simulink model "pfb_fir_generic_async_test_sim4"  (R2012b)
settings: Solver=VariableStepDiscrete  StartTime=0.0  StopTime=10.0  RelTol=1e-3
model workspace (MAT data in the model file):
  synci = [0 1 2 3 4 5 6 7 8 9 10 11 ... (131074 elements, 65537x2)]
  din0 = [0 1 2 3 4 5 6 7 8 9 10 11 ... (16386 elements, 8193x2)]
  din1 = [0 1 2 3 4 5 6 7 8 9 10 11 ... (16386 elements, 8193x2)]
  din2 = [0 1 2 3 4 5 6 7 8 9 10 11 ... (16386 elements, 8193x2)]
  din3 = [0 1 2 3 4 5 6 7 8 9 10 11 ... (16386 elements, 8193x2)]
  din4 = [0 1 2 3 4 5 6 7 8 9 10 11 ... (16386 elements, 8193x2)]
  din5 = [0 1 2 3 4 5 6 7 8 9 10 11 ... (16386 elements, 8193x2)]
  din6 = [0 1 2 3 4 5 6 7 8 9 10 11 ... (16386 elements, 8193x2)]
  din7 = [0 1 2 3 4 5 6 7 8 9 10 11 ... (16386 elements, 8193x2)]
  dvalid = [0 1 2 3 4 5 6 7 8 9 10 11 ... (131072 elements, 65536x2)]
libraries: xbsIndex_r4 x3718, casper_library_delays x1
(part 10 of 18)

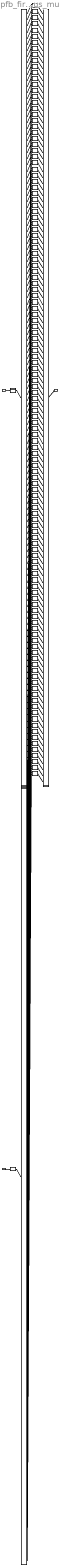
== system pfb_fir_generic_async_test_sim4/pfb_fir_generic/pfb_fir_taps/bus_mult ==
  a : Inport
  b : Inport  Port=2
  a*b_bussify : Subsystem  AncestorBlock=casper_library_flow_control/bus_create  mask(bus_create){inputNum=128}
      mask prompts: inputNum "Number of inputs:"
      mask init:
      | bus_create_init(gcb,...
      |     'inputNum', inputNum);
  a_debus : Subsystem  AncestorBlock=casper_library_flow_control/bus_expand  mask(bus_expand){mode=divisions of arbitrary size, outputNum=1, outputWidth=[10 10 10 10 10 10 10 10 10 10 10 10 10 10 10 10 10 10 10 10 10 10 10 10 10 10 10 10 10 10 10 10 10 10 10 10 10 10 10 10 10 10 10 10 10 10 10 10 10 10 10 10 10 10 10 10 10 10 10 10 10 10 10 10 10 10 10 10 10 10 10 10 10 10 10 10 10 10 10 10 10 10 10 10 10 10 10 10 10 10 10 10 10 10 10 10 10 10 10 10 10 10 10 10 10 10 10 10 10 10 10 10 10 10 10 10 10 10 10 10 10 10 10 10 10 10 10 10], outputBinaryPt=[9 9 9 9 9 9 9 9 9 9 9 9 9 9 9 9 9 9 9 9 9 9 9 9 9 9 9 9 9 9 9 9 9 9 9 9 9 9 9 9 9 9 9 9 9 9 9 9 9 9 9 9 9 9 9 9 9 9 9 9 9 9 9 9 9 9 9 9 9 9 9 9 9 9 9 9 9 9 9 9 9 9 9 9 9 9 9 9 9 9 9 9 9 9 9 9 9 9 9 9 9 9 9 9 9 9 9 9 9 9 9 9 9 9 9 9 9 9 9 9 9 9 9 9 9 9 9 9], outputArithmeticType=[1 1 1 1 1 1 1 1 1 1 1 1 1 1 1 1 1 1 1 1 1 1 1 1 1 1 1 1 1 1 1 1 1 1 1 1 1 1 1 1 1 1 1 1 1 1 1 1 1 1 1 1 1 1 1 1 1 1 1 1 1 1 1 1 1 1 1 1 1 1 1 1 1 1 1 1 1 1 1 1 1 1 1 1 1 1 1 1 1 1 1 1 1 1 1 1 1 1 1 1 1 1 1 1 1 1 1 1 1 1 1 1 1 1 1 1 1 1 1 1 1 1 1 1 1 1 1 1], show_format=on, outputToWorkspace=off, variablePrefix=, outputToModelAsWell=on}
      mask prompts: outputNum "Number of outputs:"; outputWidth "Output width [msb ... lsb]:"; outputBinaryPt "Output binary point position [msb ... lsb]:"; outputArithmeticType "Output arithmetic type (ufix=0, fix=1, bool=2) [msb ... lsb]:"; show_format "Print format string?"; outputToWorkspace "Output to workspace?"; variablePrefix "Variable name prefix:"; outputToModelAsWell "Output to model as well?"
      mask help:
      | Expands a 'bus' made using a bus_create or Xilinx
      | concat block.
      | The input will be divided into the specified number
      | of outputs with the specified arithmetic types.
      | Divisions are made from most significant bit.
      mask init: same as pfb_fir_generic_async_test_sim4/pfb_fir_generic/bus_expand
      settings: AttributesFormatString=128 outputs: f10.9,f10.9,f10.9,f10.9,f10.9,f10.9,f10.9,f10.9,f10.9,f10.9,f10.9,f10.9,f10.9,f10.9,f10.9,f10.9,f10.9,f10.9,f10.9,f10.9,f10.9,f10.9,f10.9,f10.9,f10.9,f10.9,f10.9,f10.9,f10.9,f10.9,f10.9,f10.9,f10.9,f10.9,f10.9,f10.9,f10.9,f10.9,f10.9,f10.9,f10.9,f10.9,f10.9,f10.9,f10.9,f10.9,f10.9,f10.9,f10.9,f10.9,f10.9,f10.9,f10.9,f10.9,f10.9,f10.9,f10.9,f10.9,f10.9,f10.9,f10.9,f10.9,f10.9,f10.9,f10.9,f10.9,f10.9,f10.9,f10.9,f10.9,f10.9,f10.9,f10.9,f10.9,f10.9,f10.9,f10.9,f10.9,f10.9,f10.9,f10.9,f10.9,f10.9,f10.9,f10.9,f10.9,f10.9,f10.9,f10.9,f10.9,f10.9,f10.9,f10.9,f10.9,f10.9,f10.9,f10.9,f10.9,f10.9,f10.9,f10.9,f10.9,f10.9,f10.9,f10.9,f10.9,f10.9,f10.9,f10.9,f10.9,f10.9,f10.9,f10.9,f10.9,f10.9,f10.9,f10.9,f10.9,f10.9,f10.9,f10.9,f10.9,f10.9,f10.9,f10.9,f10.9,f10.9,f10.9,
      mask TypeOptions mode: divisions of equal size | divisions of arbitrary size
      mask Callback mode: bus_expand_callback();
      mask Callback outputWidth: bus_expand_callback();
      mask Callback outputToWorkspace: bus_expand_callback();
  b_debus : Subsystem  AncestorBlock=casper_library_flow_control/bus_expand  mask(bus_expand){mode=divisions of arbitrary size, outputNum=1, outputWidth=[18 18 18 18 18 18 18 18 18 18 18 18 18 18 18 18 18 18 18 18 18 18 18 18 18 18 18 18 18 18 18 18 18 18 18 18 18 18 18 18 18 18 18 18 18 18 18 18 18 18 18 18 18 18 18 18 18 18 18 18 18 18 18 18 18 18 18 18 18 18 18 18 18 18 18 18 18 18 18 18 18 18 18 18 18 18 18 18 18 18 18 18 18 18 18 18 18 18 18 18 18 18 18 18 18 18 18 18 18 18 18 18 18 18 18 18 18 18 18 18 18 18 18 18 18 18 18 18], outputBinaryPt=[17 17 17 17 17 17 17 17 17 17 17 17 17 17 17 17 17 17 17 17 17 17 17 17 17 17 17 17 17 17 17 17 17 17 17 17 17 17 17 17 17 17 17 17 17 17 17 17 17 17 17 17 17 17 17 17 17 17 17 17 17 17 17 17 17 17 17 17 17 17 17 17 17 17 17 17 17 17 17 17 17 17 17 17 17 17 17 17 17 17 17 17 17 17 17 17 17 17 17 17 17 17 17 17 17 17 17 17 17 17 17 17 17 17 17 17 17 17 17 17 17 17 17 17 17 17 17 17], outputArithmeticType=[1 1 1 1 1 1 1 1 1 1 1 1 1 1 1 1 1 1 1 1 1 1 1 1 1 1 1 1 1 1 1 1 1 1 1 1 1 1 1 1 1 1 1 1 1 1 1 1 1 1 1 1 1 1 1 1 1 1 1 1 1 1 1 1 1 1 1 1 1 1 1 1 1 1 1 1 1 1 1 1 1 1 1 1 1 1 1 1 1 1 1 1 1 1 1 1 1 1 1 1 1 1 1 1 1 1 1 1 1 1 1 1 1 1 1 1 1 1 1 1 1 1 1 1 1 1 1 1], show_format=on, outputToWorkspace=off, variablePrefix=, outputToModelAsWell=on}
      mask prompts: outputNum "Number of outputs:"; outputWidth "Output width [msb ... lsb]:"; outputBinaryPt "Output binary point position [msb ... lsb]:"; outputArithmeticType "Output arithmetic type (ufix=0, fix=1, bool=2) [msb ... lsb]:"; show_format "Print format string?"; outputToWorkspace "Output to workspace?"; variablePrefix "Variable name prefix:"; outputToModelAsWell "Output to model as well?"
      mask help:
      | Expands a 'bus' made using a bus_create or Xilinx
      | concat block.
      | The input will be divided into the specified number
      | of outputs with the specified arithmetic types.
      | Divisions are made from most significant bit.
      mask init: same as pfb_fir_generic_async_test_sim4/pfb_fir_generic/bus_expand
      settings: AttributesFormatString=128 outputs: f18.17,f18.17,f18.17,f18.17,f18.17,f18.17,f18.17,f18.17,f18.17,f18.17,f18.17,f18.17,f18.17,f18.17,f18.17,f18.17,f18.17,f18.17,f18.17,f18.17,f18.17,f18.17,f18.17,f18.17,f18.17,f18.17,f18.17,f18.17,f18.17,f18.17,f18.17,f18.17,f18.17,f18.17,f18.17,f18.17,f18.17,f18.17,f18.17,f18.17,f18.17,f18.17,f18.17,f18.17,f18.17,f18.17,f18.17,f18.17,f18.17,f18.17,f18.17,f18.17,f18.17,f18.17,f18.17,f18.17,f18.17,f18.17,f18.17,f18.17,f18.17,f18.17,f18.17,f18.17,f18.17,f18.17,f18.17,f18.17,f18.17,f18.17,f18.17,f18.17,f18.17,f18.17,f18.17,f18.17,f18.17,f18.17,f18.17,f18.17,f18.17,f18.17,f18.17,f18.17,f18.17,f18.17,f18.17,f18.17,f18.17,f18.17,f18.17,f18.17,f18.17,f18.17,f18.17,f18.17,f18.17,f18.17,f18.17,f18.17,f18.17,f18.17,f18.17,f18.17,f18.17,f18.17,f18.17,f18.17,f18.17,f18.17,f18.17,f18.17,f18.17,f18.17,f18.17,f18.17,f18.17,f18.17,f18.17,f18.17,f18.17,f18.17,f18.17,f18.17,f18.17,f18.17,f18.17,f18.17,
      mask TypeOptions mode: divisions of equal size | divisions of arbitrary size
      mask Callback mode: bus_expand_callback();
      mask Callback outputWidth: bus_expand_callback();
      mask Callback outputToWorkspace: bus_expand_callback();
  mult{1..128} (128 alike) : xbsIndex_r4/Mult  precision=User Defined  arith_type="Signed  (2's comp)"  n_bits=28  bin_pt=26  quantization=Truncate  overflow=Wrap  en=off  latency=mult_latency  dbl_ovrd=off  use_behavioral_HDL=on  opt=Speed  use_embedded=off  optimum_pipeline=off  pipeline=on  use_rpm=on  placement_style=Triangular  block_type=mult
  repa : Subsystem  AncestorBlock=casper_library_bus/bus_replicate  mask(bus_replicate){replication=1, latency=0, misc=off, implementation=core}
      mask prompts: replication "replication factor"; misc "misc support"; implementation "delay implementation"
      mask help: Output bus formed by replicating input bus a number of times
      mask init:
      | bus_replicate_init(gcb, ...
      |     'replication', replication, ...
      |     'latency', latency, ...
      |     'implementation', implementation, ...
      |     'misc', misc);
      mask TypeOptions implementation: core | behavioral
  repb : Subsystem  AncestorBlock=casper_library_bus/bus_replicate  mask(bus_replicate){replication=1, latency=0, misc=off, implementation=core}
      mask prompts: replication "replication factor"; misc "misc support"; implementation "delay implementation"
      mask help: Output bus formed by replicating input bus a number of times
      mask init:
      | bus_replicate_init(gcb, ...
      |     'replication', replication, ...
      |     'latency', latency, ...
      |     'implementation', implementation, ...
      |     'misc', misc);
      mask TypeOptions implementation: core | behavioral
  a*b : Outport
  wires:
  a/1 -> repa/1(in)
  b/1 -> repb/1(in)
  repa/1(out) -> a_debus/1(bus_in)
  repb/1(out) -> b_debus/1(bus_in)
  a_debus/1(msb_out128) -> mult1/1
  b_debus/1(msb_out128) -> mult1/2
  a_debus/2(out127) -> mult2/1
  b_debus/2(out127) -> mult2/2
  a_debus/3(out126) -> mult3/1
  b_debus/3(out126) -> mult3/2
  a_debus/4(out125) -> mult4/1
  b_debus/4(out125) -> mult4/2
  a_debus/5(out124) -> mult5/1
  b_debus/5(out124) -> mult5/2
  a_debus/6(out123) -> mult6/1
  b_debus/6(out123) -> mult6/2
  a_debus/7(out122) -> mult7/1
  b_debus/7(out122) -> mult7/2
  a_debus/8(out121) -> mult8/1
  b_debus/8(out121) -> mult8/2
  a_debus/9(out120) -> mult9/1
  b_debus/9(out120) -> mult9/2
  a_debus/10(out119) -> mult10/1
  b_debus/10(out119) -> mult10/2
  a_debus/11(out118) -> mult11/1
  b_debus/11(out118) -> mult11/2
  a_debus/12(out117) -> mult12/1
  b_debus/12(out117) -> mult12/2
  a_debus/13(out116) -> mult13/1
  b_debus/13(out116) -> mult13/2
  a_debus/14(out115) -> mult14/1
  b_debus/14(out115) -> mult14/2
  a_debus/15(out114) -> mult15/1
  b_debus/15(out114) -> mult15/2
  a_debus/16(out113) -> mult16/1
  b_debus/16(out113) -> mult16/2
  a_debus/17(out112) -> mult17/1
  b_debus/17(out112) -> mult17/2
  a_debus/18(out111) -> mult18/1
  b_debus/18(out111) -> mult18/2
  a_debus/19(out110) -> mult19/1
  b_debus/19(out110) -> mult19/2
  a_debus/20(out109) -> mult20/1
  b_debus/20(out109) -> mult20/2
  a_debus/21(out108) -> mult21/1
  b_debus/21(out108) -> mult21/2
  a_debus/22(out107) -> mult22/1
  b_debus/22(out107) -> mult22/2
  a_debus/23(out106) -> mult23/1
  b_debus/23(out106) -> mult23/2
  a_debus/24(out105) -> mult24/1
  b_debus/24(out105) -> mult24/2
  a_debus/25(out104) -> mult25/1
  b_debus/25(out104) -> mult25/2
  a_debus/26(out103) -> mult26/1
  b_debus/26(out103) -> mult26/2
  a_debus/27(out102) -> mult27/1
  b_debus/27(out102) -> mult27/2
  a_debus/28(out101) -> mult28/1
  b_debus/28(out101) -> mult28/2
  a_debus/29(out100) -> mult29/1
  b_debus/29(out100) -> mult29/2
  a_debus/30(out99) -> mult30/1
  b_debus/30(out99) -> mult30/2
  a_debus/31(out98) -> mult31/1
  b_debus/31(out98) -> mult31/2
  a_debus/32(out97) -> mult32/1
  b_debus/32(out97) -> mult32/2
  a_debus/33(out96) -> mult33/1
  b_debus/33(out96) -> mult33/2
  a_debus/34(out95) -> mult34/1
  b_debus/34(out95) -> mult34/2
  a_debus/35(out94) -> mult35/1
  b_debus/35(out94) -> mult35/2
  a_debus/36(out93) -> mult36/1
  b_debus/36(out93) -> mult36/2
  a_debus/37(out92) -> mult37/1
  b_debus/37(out92) -> mult37/2
  a_debus/38(out91) -> mult38/1
  b_debus/38(out91) -> mult38/2
  a_debus/39(out90) -> mult39/1
  b_debus/39(out90) -> mult39/2
  a_debus/40(out89) -> mult40/1
  b_debus/40(out89) -> mult40/2
  a_debus/41(out88) -> mult41/1
  b_debus/41(out88) -> mult41/2
  a_debus/42(out87) -> mult42/1
  b_debus/42(out87) -> mult42/2
  a_debus/43(out86) -> mult43/1
  b_debus/43(out86) -> mult43/2
  a_debus/44(out85) -> mult44/1
  b_debus/44(out85) -> mult44/2
  a_debus/45(out84) -> mult45/1
  b_debus/45(out84) -> mult45/2
  a_debus/46(out83) -> mult46/1
  b_debus/46(out83) -> mult46/2
  a_debus/47(out82) -> mult47/1
  b_debus/47(out82) -> mult47/2
  a_debus/48(out81) -> mult48/1
  b_debus/48(out81) -> mult48/2
  a_debus/49(out80) -> mult49/1
  b_debus/49(out80) -> mult49/2
  a_debus/50(out79) -> mult50/1
  b_debus/50(out79) -> mult50/2
  a_debus/51(out78) -> mult51/1
  b_debus/51(out78) -> mult51/2
  a_debus/52(out77) -> mult52/1
  b_debus/52(out77) -> mult52/2
  a_debus/53(out76) -> mult53/1
  b_debus/53(out76) -> mult53/2
  a_debus/54(out75) -> mult54/1
  b_debus/54(out75) -> mult54/2
  a_debus/55(out74) -> mult55/1
  b_debus/55(out74) -> mult55/2
  a_debus/56(out73) -> mult56/1
  b_debus/56(out73) -> mult56/2
  a_debus/57(out72) -> mult57/1
  b_debus/57(out72) -> mult57/2
  a_debus/58(out71) -> mult58/1
  b_debus/58(out71) -> mult58/2
  a_debus/59(out70) -> mult59/1
  b_debus/59(out70) -> mult59/2
  a_debus/60(out69) -> mult60/1
  b_debus/60(out69) -> mult60/2
  a_debus/61(out68) -> mult61/1
  b_debus/61(out68) -> mult61/2
  a_debus/62(out67) -> mult62/1
  b_debus/62(out67) -> mult62/2
  a_debus/63(out66) -> mult63/1
  b_debus/63(out66) -> mult63/2
  a_debus/64(out65) -> mult64/1
  b_debus/64(out65) -> mult64/2
  a_debus/65(out64) -> mult65/1
  b_debus/65(out64) -> mult65/2
  a_debus/66(out63) -> mult66/1
  b_debus/66(out63) -> mult66/2
  a_debus/67(out62) -> mult67/1
  b_debus/67(out62) -> mult67/2
  a_debus/68(out61) -> mult68/1
  b_debus/68(out61) -> mult68/2
  a_debus/69(out60) -> mult69/1
  b_debus/69(out60) -> mult69/2
  a_debus/70(out59) -> mult70/1
  b_debus/70(out59) -> mult70/2
  a_debus/71(out58) -> mult71/1
  b_debus/71(out58) -> mult71/2
  a_debus/72(out57) -> mult72/1
  b_debus/72(out57) -> mult72/2
  a_debus/73(out56) -> mult73/1
  b_debus/73(out56) -> mult73/2
  a_debus/74(out55) -> mult74/1
  b_debus/74(out55) -> mult74/2
  a_debus/75(out54) -> mult75/1
  b_debus/75(out54) -> mult75/2
  a_debus/76(out53) -> mult76/1
  b_debus/76(out53) -> mult76/2
  a_debus/77(out52) -> mult77/1
  b_debus/77(out52) -> mult77/2
  a_debus/78(out51) -> mult78/1
  b_debus/78(out51) -> mult78/2
  a_debus/79(out50) -> mult79/1
  b_debus/79(out50) -> mult79/2
  a_debus/80(out49) -> mult80/1
  b_debus/80(out49) -> mult80/2
  a_debus/81(out48) -> mult81/1
  b_debus/81(out48) -> mult81/2
  a_debus/82(out47) -> mult82/1
  b_debus/82(out47) -> mult82/2
  a_debus/83(out46) -> mult83/1
  b_debus/83(out46) -> mult83/2
  a_debus/84(out45) -> mult84/1
  b_debus/84(out45) -> mult84/2
  a_debus/85(out44) -> mult85/1
  b_debus/85(out44) -> mult85/2
  a_debus/86(out43) -> mult86/1
  b_debus/86(out43) -> mult86/2
  a_debus/87(out42) -> mult87/1
  b_debus/87(out42) -> mult87/2
  a_debus/88(out41) -> mult88/1
  b_debus/88(out41) -> mult88/2
  a_debus/89(out40) -> mult89/1
  b_debus/89(out40) -> mult89/2
  a_debus/90(out39) -> mult90/1
  b_debus/90(out39) -> mult90/2
  a_debus/91(out38) -> mult91/1
  b_debus/91(out38) -> mult91/2
  a_debus/92(out37) -> mult92/1
  b_debus/92(out37) -> mult92/2
  a_debus/93(out36) -> mult93/1
  b_debus/93(out36) -> mult93/2
  a_debus/94(out35) -> mult94/1
  b_debus/94(out35) -> mult94/2
  a_debus/95(out34) -> mult95/1
  b_debus/95(out34) -> mult95/2
  a_debus/96(out33) -> mult96/1
  b_debus/96(out33) -> mult96/2
  a_debus/97(out32) -> mult97/1
  b_debus/97(out32) -> mult97/2
  a_debus/98(out31) -> mult98/1
  b_debus/98(out31) -> mult98/2
  a_debus/99(out30) -> mult99/1
  b_debus/99(out30) -> mult99/2
  a_debus/100(out29) -> mult100/1
  b_debus/100(out29) -> mult100/2
  a_debus/101(out28) -> mult101/1
  b_debus/101(out28) -> mult101/2
  a_debus/102(out27) -> mult102/1
  b_debus/102(out27) -> mult102/2
  a_debus/103(out26) -> mult103/1
  b_debus/103(out26) -> mult103/2
  a_debus/104(out25) -> mult104/1
  b_debus/104(out25) -> mult104/2
  a_debus/105(out24) -> mult105/1
  b_debus/105(out24) -> mult105/2
  a_debus/106(out23) -> mult106/1
  b_debus/106(out23) -> mult106/2
  a_debus/107(out22) -> mult107/1
  b_debus/107(out22) -> mult107/2
  a_debus/108(out21) -> mult108/1
  b_debus/108(out21) -> mult108/2
  a_debus/109(out20) -> mult109/1
  b_debus/109(out20) -> mult109/2
  a_debus/110(out19) -> mult110/1
  b_debus/110(out19) -> mult110/2
  a_debus/111(out18) -> mult111/1
  b_debus/111(out18) -> mult111/2
  a_debus/112(out17) -> mult112/1
  b_debus/112(out17) -> mult112/2
  a_debus/113(out16) -> mult113/1
  b_debus/113(out16) -> mult113/2
  a_debus/114(out15) -> mult114/1
  b_debus/114(out15) -> mult114/2
  a_debus/115(out14) -> mult115/1
  b_debus/115(out14) -> mult115/2
  a_debus/116(out13) -> mult116/1
  b_debus/116(out13) -> mult116/2
  a_debus/117(out12) -> mult117/1
  b_debus/117(out12) -> mult117/2
  a_debus/118(out11) -> mult118/1
  b_debus/118(out11) -> mult118/2
  a_debus/119(out10) -> mult119/1
  b_debus/119(out10) -> mult119/2
  a_debus/120(out9) -> mult120/1
  b_debus/120(out9) -> mult120/2
  a_debus/121(out8) -> mult121/1
  b_debus/121(out8) -> mult121/2
  a_debus/122(out7) -> mult122/1
  b_debus/122(out7) -> mult122/2
  a_debus/123(out6) -> mult123/1
  b_debus/123(out6) -> mult123/2
  a_debus/124(out5) -> mult124/1
  b_debus/124(out5) -> mult124/2
  a_debus/125(out4) -> mult125/1
  b_debus/125(out4) -> mult125/2
  a_debus/126(out3) -> mult126/1
  b_debus/126(out3) -> mult126/2
  a_debus/127(out2) -> mult127/1
  b_debus/127(out2) -> mult127/2
  a_debus/128(lsb_out1) -> mult128/1
  b_debus/128(lsb_out1) -> mult128/2
  mult1/1 -> a*b_bussify/1(in1)
  mult2/1 -> a*b_bussify/2(in2)
  mult3/1 -> a*b_bussify/3(in3)
  mult4/1 -> a*b_bussify/4(in4)
  mult5/1 -> a*b_bussify/5(in5)
  mult6/1 -> a*b_bussify/6(in6)
  mult7/1 -> a*b_bussify/7(in7)
  mult8/1 -> a*b_bussify/8(in8)
  mult9/1 -> a*b_bussify/9(in9)
  mult10/1 -> a*b_bussify/10(in10)
  mult11/1 -> a*b_bussify/11(in11)
  mult12/1 -> a*b_bussify/12(in12)
  mult13/1 -> a*b_bussify/13(in13)
  mult14/1 -> a*b_bussify/14(in14)
  mult15/1 -> a*b_bussify/15(in15)
  mult16/1 -> a*b_bussify/16(in16)
  mult17/1 -> a*b_bussify/17(in17)
  mult18/1 -> a*b_bussify/18(in18)
  mult19/1 -> a*b_bussify/19(in19)
  mult20/1 -> a*b_bussify/20(in20)
  mult21/1 -> a*b_bussify/21(in21)
  mult22/1 -> a*b_bussify/22(in22)
  mult23/1 -> a*b_bussify/23(in23)
  mult24/1 -> a*b_bussify/24(in24)
  mult25/1 -> a*b_bussify/25(in25)
  mult26/1 -> a*b_bussify/26(in26)
  mult27/1 -> a*b_bussify/27(in27)
  mult28/1 -> a*b_bussify/28(in28)
  mult29/1 -> a*b_bussify/29(in29)
  mult30/1 -> a*b_bussify/30(in30)
  mult31/1 -> a*b_bussify/31(in31)
  mult32/1 -> a*b_bussify/32(in32)
  mult33/1 -> a*b_bussify/33(in33)
  mult34/1 -> a*b_bussify/34(in34)
  mult35/1 -> a*b_bussify/35(in35)
  mult36/1 -> a*b_bussify/36(in36)
  mult37/1 -> a*b_bussify/37(in37)
  mult38/1 -> a*b_bussify/38(in38)
  mult39/1 -> a*b_bussify/39(in39)
  mult40/1 -> a*b_bussify/40(in40)
  mult41/1 -> a*b_bussify/41(in41)
  mult42/1 -> a*b_bussify/42(in42)
  mult43/1 -> a*b_bussify/43(in43)
  mult44/1 -> a*b_bussify/44(in44)
  mult45/1 -> a*b_bussify/45(in45)
  mult46/1 -> a*b_bussify/46(in46)
  mult47/1 -> a*b_bussify/47(in47)
  mult48/1 -> a*b_bussify/48(in48)
  mult49/1 -> a*b_bussify/49(in49)
  mult50/1 -> a*b_bussify/50(in50)
  mult51/1 -> a*b_bussify/51(in51)
  mult52/1 -> a*b_bussify/52(in52)
  mult53/1 -> a*b_bussify/53(in53)
  mult54/1 -> a*b_bussify/54(in54)
  mult55/1 -> a*b_bussify/55(in55)
  mult56/1 -> a*b_bussify/56(in56)
  mult57/1 -> a*b_bussify/57(in57)
  mult58/1 -> a*b_bussify/58(in58)
  mult59/1 -> a*b_bussify/59(in59)
  mult60/1 -> a*b_bussify/60(in60)
  mult61/1 -> a*b_bussify/61(in61)
  mult62/1 -> a*b_bussify/62(in62)
  mult63/1 -> a*b_bussify/63(in63)
  mult64/1 -> a*b_bussify/64(in64)
  mult65/1 -> a*b_bussify/65(in65)
  mult66/1 -> a*b_bussify/66(in66)
  mult67/1 -> a*b_bussify/67(in67)
  mult68/1 -> a*b_bussify/68(in68)
  mult69/1 -> a*b_bussify/69(in69)
  mult70/1 -> a*b_bussify/70(in70)
  mult71/1 -> a*b_bussify/71(in71)
  mult72/1 -> a*b_bussify/72(in72)
  mult73/1 -> a*b_bussify/73(in73)
  mult74/1 -> a*b_bussify/74(in74)
  mult75/1 -> a*b_bussify/75(in75)
  mult76/1 -> a*b_bussify/76(in76)
  mult77/1 -> a*b_bussify/77(in77)
  mult78/1 -> a*b_bussify/78(in78)
  mult79/1 -> a*b_bussify/79(in79)
  mult80/1 -> a*b_bussify/80(in80)
  mult81/1 -> a*b_bussify/81(in81)
  mult82/1 -> a*b_bussify/82(in82)
  mult83/1 -> a*b_bussify/83(in83)
  mult84/1 -> a*b_bussify/84(in84)
  mult85/1 -> a*b_bussify/85(in85)
  mult86/1 -> a*b_bussify/86(in86)
  mult87/1 -> a*b_bussify/87(in87)
  mult88/1 -> a*b_bussify/88(in88)
  mult89/1 -> a*b_bussify/89(in89)
  mult90/1 -> a*b_bussify/90(in90)
  mult91/1 -> a*b_bussify/91(in91)
  mult92/1 -> a*b_bussify/92(in92)
  mult93/1 -> a*b_bussify/93(in93)
  mult94/1 -> a*b_bussify/94(in94)
  mult95/1 -> a*b_bussify/95(in95)
  mult96/1 -> a*b_bussify/96(in96)
  mult97/1 -> a*b_bussify/97(in97)
  mult98/1 -> a*b_bussify/98(in98)
  mult99/1 -> a*b_bussify/99(in99)
  mult100/1 -> a*b_bussify/100(in100)
  mult101/1 -> a*b_bussify/101(in101)
  mult102/1 -> a*b_bussify/102(in102)
  mult103/1 -> a*b_bussify/103(in103)
  mult104/1 -> a*b_bussify/104(in104)
  mult105/1 -> a*b_bussify/105(in105)
  mult106/1 -> a*b_bussify/106(in106)
  mult107/1 -> a*b_bussify/107(in107)
  mult108/1 -> a*b_bussify/108(in108)
  mult109/1 -> a*b_bussify/109(in109)
  mult110/1 -> a*b_bussify/110(in110)
  mult111/1 -> a*b_bussify/111(in111)
  mult112/1 -> a*b_bussify/112(in112)
  mult113/1 -> a*b_bussify/113(in113)
  mult114/1 -> a*b_bussify/114(in114)
  mult115/1 -> a*b_bussify/115(in115)
  mult116/1 -> a*b_bussify/116(in116)
  mult117/1 -> a*b_bussify/117(in117)
  mult118/1 -> a*b_bussify/118(in118)
  mult119/1 -> a*b_bussify/119(in119)
  mult120/1 -> a*b_bussify/120(in120)
  mult121/1 -> a*b_bussify/121(in121)
  mult122/1 -> a*b_bussify/122(in122)
  mult123/1 -> a*b_bussify/123(in123)
  mult124/1 -> a*b_bussify/124(in124)
  mult125/1 -> a*b_bussify/125(in125)
  mult126/1 -> a*b_bussify/126(in126)
  mult127/1 -> a*b_bussify/127(in127)
  mult128/1 -> a*b_bussify/128(in128)
  a*b_bussify/1(bus_out) -> a*b/1

== system pfb_fir_generic_async_test_sim4/pfb_fir_generic/pfb_fir_taps/tap_delays ==
  addra : Inport
  dina : Inport  Port=2
  wea : Inport  Port=3
  addrb : Inport  Port=4
  dinb : Inport  Port=5
  web : Inport  Port=6
  A_bussify : Subsystem  AncestorBlock=casper_library_flow_control/bus_create  mask(bus_create){inputNum=32}
      mask prompts: inputNum "Number of inputs:"
      mask init:
      | bus_create_init(gcb,...
      |     'inputNum', inputNum);
  B_bussify : Subsystem  AncestorBlock=casper_library_flow_control/bus_create  mask(bus_create){inputNum=32}
      mask prompts: inputNum "Number of inputs:"
      mask init:
      | bus_create_init(gcb,...
      |     'inputNum', inputNum);
  bram{0..31} (32 alike) : xbsIndex_r4/Dual Port RAM  depth=1024  initVector=getfield(get_param(gcb, 'UserData'), 'initVector')  distributed_mem=Block RAM  init_a=0  init_b=0  rst_a=off  rst_b=off  en_a=off  en_b=off  latency=8  write_mode_A=Read Before Write  write_mode_B=Read Before Write  dbl_ovrd=off  optimize=Speed  block_type=dpram
  ddina : xbsIndex_r4/Delay  rst=off  infoeditControl=Selection of Reset will increase slice count due to use of real FFs and instead of SRLs  en=off  latency=0  dbl_ovrd=off  reg_retiming=on  block_type=delay
  ddinb : xbsIndex_r4/Delay  rst=off  infoeditControl=Selection of Reset will increase slice count due to use of real FFs and instead of SRLs  en=off  latency=9  dbl_ovrd=off  reg_retiming=off  block_type=delay
  debus_addra : Subsystem  AncestorBlock=casper_library_flow_control/bus_expand  mask(bus_expand){mode=divisions of equal size, outputNum=32, outputWidth=[10 10 10 10 10 10 10 10 10 10 10 10 10 10 10 10 10 10 10 10 10 10 10 10 10 10 10 10 10 10 10 10], outputBinaryPt=[0 0 0 0 0 0 0 0 0 0 0 0 0 0 0 0 0 0 0 0 0 0 0 0 0 0 0 0 0 0 0 0], outputArithmeticType=[0 0 0 0 0 0 0 0 0 0 0 0 0 0 0 0 0 0 0 0 0 0 0 0 0 0 0 0 0 0 0 0], show_format=on, outputToWorkspace=off, variablePrefix=, outputToModelAsWell=on}
      mask prompts: outputNum "Number of outputs:"; outputWidth "Output width:"; outputBinaryPt "Output binary point position:"; outputArithmeticType "Output arithmetic type (ufix=0, fix=1, bool=2):"; show_format "Print format string?"; outputToWorkspace "Output to workspace?"; variablePrefix "Variable name prefix:"; outputToModelAsWell "Output to model as well?"
      mask help:
      | Expands a 'bus' made using a bus_create or Xilinx
      | concat block.
      | The input will be divided into the specified number
      | of outputs with the specified arithmetic types.
      | Divisions are made from most significant bit.
      mask init: same as pfb_fir_generic_async_test_sim4/pfb_fir_generic/bus_expand
      settings: AttributesFormatString=32 outputs: uf10.0,uf10.0,uf10.0,uf10.0,uf10.0,uf10.0,uf10.0,uf10.0,uf10.0,uf10.0,uf10.0,uf10.0,uf10.0,uf10.0,uf10.0,uf10.0,uf10.0,uf10.0,uf10.0,uf10.0,uf10.0,uf10.0,uf10.0,uf10.0,uf10.0,uf10.0,uf10.0,uf10.0,uf10.0,uf10.0,uf10.0,uf10.0,
      mask TypeOptions mode: divisions of equal size | divisions of arbitrary size
      mask Callback mode: bus_expand_callback();
      mask Callback outputWidth: bus_expand_callback();
      mask Callback outputToWorkspace: bus_expand_callback();
  debus_addrb : Subsystem  AncestorBlock=casper_library_flow_control/bus_expand  mask(bus_expand){mode=divisions of equal size, outputNum=32, outputWidth=[10 10 10 10 10 10 10 10 10 10 10 10 10 10 10 10 10 10 10 10 10 10 10 10 10 10 10 10 10 10 10 10], outputBinaryPt=[0 0 0 0 0 0 0 0 0 0 0 0 0 0 0 0 0 0 0 0 0 0 0 0 0 0 0 0 0 0 0 0], outputArithmeticType=[0 0 0 0 0 0 0 0 0 0 0 0 0 0 0 0 0 0 0 0 0 0 0 0 0 0 0 0 0 0 0 0], show_format=on, outputToWorkspace=off, variablePrefix=, outputToModelAsWell=on}
      mask prompts: outputNum "Number of outputs:"; outputWidth "Output width:"; outputBinaryPt "Output binary point position:"; outputArithmeticType "Output arithmetic type (ufix=0, fix=1, bool=2):"; show_format "Print format string?"; outputToWorkspace "Output to workspace?"; variablePrefix "Variable name prefix:"; outputToModelAsWell "Output to model as well?"
      mask help:
      | Expands a 'bus' made using a bus_create or Xilinx
      | concat block.
      | The input will be divided into the specified number
      | of outputs with the specified arithmetic types.
      | Divisions are made from most significant bit.
      mask init: same as pfb_fir_generic_async_test_sim4/pfb_fir_generic/bus_expand
      settings: AttributesFormatString=32 outputs: uf10.0,uf10.0,uf10.0,uf10.0,uf10.0,uf10.0,uf10.0,uf10.0,uf10.0,uf10.0,uf10.0,uf10.0,uf10.0,uf10.0,uf10.0,uf10.0,uf10.0,uf10.0,uf10.0,uf10.0,uf10.0,uf10.0,uf10.0,uf10.0,uf10.0,uf10.0,uf10.0,uf10.0,uf10.0,uf10.0,uf10.0,uf10.0,
      mask TypeOptions mode: divisions of equal size | divisions of arbitrary size
      mask Callback mode: bus_expand_callback();
      mask Callback outputWidth: bus_expand_callback();
      mask Callback outputToWorkspace: bus_expand_callback();
  debus_dina : Subsystem  AncestorBlock=casper_library_flow_control/bus_expand  mask(bus_expand){mode=divisions of arbitrary size, outputNum=1, outputWidth=[4 36 36 36 36 36 36 36 36 36 36 36 36 36 36 36 36 36 36 36 36 36 36 36 36 36 36 36 36 36 36 36], outputBinaryPt=[0 0 0 0 0 0 0 0 0 0 0 0 0 0 0 0 0 0 0 0 0 0 0 0 0 0 0 0 0 0 0 0], outputArithmeticType=[0 0 0 0 0 0 0 0 0 0 0 0 0 0 0 0 0 0 0 0 0 0 0 0 0 0 0 0 0 0 0 0], show_format=on, outputToWorkspace=off, variablePrefix=, outputToModelAsWell=on}
      mask prompts: outputNum "Number of outputs:"; outputWidth "Output width [msb ... lsb]:"; outputBinaryPt "Output binary point position [msb ... lsb]:"; outputArithmeticType "Output arithmetic type (ufix=0, fix=1, bool=2) [msb ... lsb]:"; show_format "Print format string?"; outputToWorkspace "Output to workspace?"; variablePrefix "Variable name prefix:"; outputToModelAsWell "Output to model as well?"
      mask help:
      | Expands a 'bus' made using a bus_create or Xilinx
      | concat block.
      | The input will be divided into the specified number
      | of outputs with the specified arithmetic types.
      | Divisions are made from most significant bit.
      mask init: same as pfb_fir_generic_async_test_sim4/pfb_fir_generic/bus_expand
      settings: AttributesFormatString=32 outputs: uf4.0,uf36.0,uf36.0,uf36.0,uf36.0,uf36.0,uf36.0,uf36.0,uf36.0,uf36.0,uf36.0,uf36.0,uf36.0,uf36.0,uf36.0,uf36.0,uf36.0,uf36.0,uf36.0,uf36.0,uf36.0,uf36.0,uf36.0,uf36.0,uf36.0,uf36.0,uf36.0,uf36.0,uf36.0,uf36.0,uf36.0,uf36.0,
      mask TypeOptions mode: divisions of equal size | divisions of arbitrary size
      mask Callback mode: bus_expand_callback();
      mask Callback outputWidth: bus_expand_callback();
      mask Callback outputToWorkspace: bus_expand_callback();
  debus_dinb : Subsystem  AncestorBlock=casper_library_flow_control/bus_expand  mask(bus_expand){mode=divisions of arbitrary size, outputNum=1, outputWidth=[4 36 36 36 36 36 36 36 36 36 36 36 36 36 36 36 36 36 36 36 36 36 36 36 36 36 36 36 36 36 36 36], outputBinaryPt=[0 0 0 0 0 0 0 0 0 0 0 0 0 0 0 0 0 0 0 0 0 0 0 0 0 0 0 0 0 0 0 0], outputArithmeticType=[0 0 0 0 0 0 0 0 0 0 0 0 0 0 0 0 0 0 0 0 0 0 0 0 0 0 0 0 0 0 0 0], show_format=on, outputToWorkspace=off, variablePrefix=, outputToModelAsWell=on}
      mask prompts: outputNum "Number of outputs:"; outputWidth "Output width [msb ... lsb]:"; outputBinaryPt "Output binary point position [msb ... lsb]:"; outputArithmeticType "Output arithmetic type (ufix=0, fix=1, bool=2) [msb ... lsb]:"; show_format "Print format string?"; outputToWorkspace "Output to workspace?"; variablePrefix "Variable name prefix:"; outputToModelAsWell "Output to model as well?"
      mask help:
      | Expands a 'bus' made using a bus_create or Xilinx
      | concat block.
      | The input will be divided into the specified number
      | of outputs with the specified arithmetic types.
      | Divisions are made from most significant bit.
      mask init: same as pfb_fir_generic_async_test_sim4/pfb_fir_generic/bus_expand
      settings: AttributesFormatString=32 outputs: uf4.0,uf36.0,uf36.0,uf36.0,uf36.0,uf36.0,uf36.0,uf36.0,uf36.0,uf36.0,uf36.0,uf36.0,uf36.0,uf36.0,uf36.0,uf36.0,uf36.0,uf36.0,uf36.0,uf36.0,uf36.0,uf36.0,uf36.0,uf36.0,uf36.0,uf36.0,uf36.0,uf36.0,uf36.0,uf36.0,uf36.0,uf36.0,
      mask TypeOptions mode: divisions of equal size | divisions of arbitrary size
      mask Callback mode: bus_expand_callback();
      mask Callback outputWidth: bus_expand_callback();
      mask Callback outputToWorkspace: bus_expand_callback();
  debus_wea : Subsystem  AncestorBlock=casper_library_flow_control/bus_expand  mask(bus_expand){mode=divisions of equal size, outputNum=32, outputWidth=[1 1 1 1 1 1 1 1 1 1 1 1 1 1 1 1 1 1 1 1 1 1 1 1 1 1 1 1 1 1 1 1], outputBinaryPt=[0 0 0 0 0 0 0 0 0 0 0 0 0 0 0 0 0 0 0 0 0 0 0 0 0 0 0 0 0 0 0 0], outputArithmeticType=[2 2 2 2 2 2 2 2 2 2 2 2 2 2 2 2 2 2 2 2 2 2 2 2 2 2 2 2 2 2 2 2], show_format=on, outputToWorkspace=off, variablePrefix=, outputToModelAsWell=on}
      mask prompts: outputNum "Number of outputs:"; outputWidth "Output width:"; outputBinaryPt "Output binary point position:"; outputArithmeticType "Output arithmetic type (ufix=0, fix=1, bool=2):"; show_format "Print format string?"; outputToWorkspace "Output to workspace?"; variablePrefix "Variable name prefix:"; outputToModelAsWell "Output to model as well?"
      mask help:
      | Expands a 'bus' made using a bus_create or Xilinx
      | concat block.
      | The input will be divided into the specified number
      | of outputs with the specified arithmetic types.
      | Divisions are made from most significant bit.
      mask init: same as pfb_fir_generic_async_test_sim4/pfb_fir_generic/bus_expand
      settings: AttributesFormatString=32 outputs: b,b,b,b,b,b,b,b,b,b,b,b,b,b,b,b,b,b,b,b,b,b,b,b,b,b,b,b,b,b,b,b,
      mask TypeOptions mode: divisions of equal size | divisions of arbitrary size
      mask Callback mode: bus_expand_callback();
      mask Callback outputWidth: bus_expand_callback();
      mask Callback outputToWorkspace: bus_expand_callback();
  debus_web : Subsystem  AncestorBlock=casper_library_flow_control/bus_expand  mask(bus_expand){mode=divisions of equal size, outputNum=32, outputWidth=[1 1 1 1 1 1 1 1 1 1 1 1 1 1 1 1 1 1 1 1 1 1 1 1 1 1 1 1 1 1 1 1], outputBinaryPt=[0 0 0 0 0 0 0 0 0 0 0 0 0 0 0 0 0 0 0 0 0 0 0 0 0 0 0 0 0 0 0 0], outputArithmeticType=[2 2 2 2 2 2 2 2 2 2 2 2 2 2 2 2 2 2 2 2 2 2 2 2 2 2 2 2 2 2 2 2], show_format=on, outputToWorkspace=off, variablePrefix=, outputToModelAsWell=on}
      mask prompts: outputNum "Number of outputs:"; outputWidth "Output width:"; outputBinaryPt "Output binary point position:"; outputArithmeticType "Output arithmetic type (ufix=0, fix=1, bool=2):"; show_format "Print format string?"; outputToWorkspace "Output to workspace?"; variablePrefix "Variable name prefix:"; outputToModelAsWell "Output to model as well?"
      mask help:
      | Expands a 'bus' made using a bus_create or Xilinx
      | concat block.
      | The input will be divided into the specified number
      | of outputs with the specified arithmetic types.
      | Divisions are made from most significant bit.
      mask init: same as pfb_fir_generic_async_test_sim4/pfb_fir_generic/bus_expand
      settings: AttributesFormatString=32 outputs: b,b,b,b,b,b,b,b,b,b,b,b,b,b,b,b,b,b,b,b,b,b,b,b,b,b,b,b,b,b,b,b,
      mask TypeOptions mode: divisions of equal size | divisions of arbitrary size
      mask Callback mode: bus_expand_callback();
      mask Callback outputWidth: bus_expand_callback();
      mask Callback outputToWorkspace: bus_expand_callback();
  rep_addra : Subsystem  AncestorBlock=casper_library_bus/bus_replicate  mask(bus_replicate){replication=32, latency=9, misc=off, implementation=core}
      mask prompts: replication "replication factor"; misc "misc support"; implementation "delay implementation"
      mask help: Output bus formed by replicating input bus a number of times
      mask init:
      | bus_replicate_init(gcb, ...
      |     'replication', replication, ...
      |     'latency', latency, ...
      |     'implementation', implementation, ...
      |     'misc', misc);
      mask TypeOptions implementation: core | behavioral
  rep_addrb : Subsystem  AncestorBlock=casper_library_bus/bus_replicate  mask(bus_replicate){replication=32, latency=9, misc=off, implementation=core}
      mask prompts: replication "replication factor"; misc "misc support"; implementation "delay implementation"
      mask help: Output bus formed by replicating input bus a number of times
      mask init:
      | bus_replicate_init(gcb, ...
      |     'replication', replication, ...
      |     'latency', latency, ...
      |     'implementation', implementation, ...
      |     'misc', misc);
      mask TypeOptions implementation: core | behavioral
  rep_wea : Subsystem  AncestorBlock=casper_library_bus/bus_replicate  mask(bus_replicate){replication=32, latency=0, misc=off, implementation=behavioral}
      mask prompts: replication "replication factor"; misc "misc support"; implementation "delay implementation"
      mask help: Output bus formed by replicating input bus a number of times
      mask init:
      | bus_replicate_init(gcb, ...
      |     'replication', replication, ...
      |     'latency', latency, ...
      |     'implementation', implementation, ...
      |     'misc', misc);
      mask TypeOptions implementation: core | behavioral
  rep_web : Subsystem  AncestorBlock=casper_library_bus/bus_replicate  mask(bus_replicate){replication=32, latency=9, misc=off, implementation=core}
      mask prompts: replication "replication factor"; misc "misc support"; implementation "delay implementation"
      mask help: Output bus formed by replicating input bus a number of times
      mask init:
      | bus_replicate_init(gcb, ...
      |     'replication', replication, ...
      |     'latency', latency, ...
      |     'implementation', implementation, ...
      |     'misc', misc);
      mask TypeOptions implementation: core | behavioral
  A : Outport
  B : Outport  Port=2
  wires:
  addra/1 -> rep_addra/1(in)
  dina/1 -> ddina/1
  wea/1 -> rep_wea/1(in)
  addrb/1 -> rep_addrb/1(in)
  dinb/1 -> ddinb/1
  web/1 -> rep_web/1(in)
  rep_addra/1(out) -> debus_addra/1(bus_in)
  ddina/1 -> debus_dina/1(bus_in)
  rep_wea/1(out) -> debus_wea/1(bus_in)
  rep_addrb/1(out) -> debus_addrb/1(bus_in)
  ddinb/1 -> debus_dinb/1(bus_in)
  rep_web/1(out) -> debus_web/1(bus_in)
  debus_addra/1(msb_out32) -> bram0/1
  debus_dina/1(msb_out32) -> bram0/2
  debus_wea/1(msb_out32) -> bram0/3
  debus_addrb/1(msb_out32) -> bram0/4
  debus_dinb/1(msb_out32) -> bram0/5
  debus_web/1(msb_out32) -> bram0/6
  debus_addra/2(out31) -> bram1/1
  debus_dina/2(out31) -> bram1/2
  debus_wea/2(out31) -> bram1/3
  debus_addrb/2(out31) -> bram1/4
  debus_dinb/2(out31) -> bram1/5
  debus_web/2(out31) -> bram1/6
  debus_addra/3(out30) -> bram2/1
  debus_dina/3(out30) -> bram2/2
  debus_wea/3(out30) -> bram2/3
  debus_addrb/3(out30) -> bram2/4
  debus_dinb/3(out30) -> bram2/5
  debus_web/3(out30) -> bram2/6
  debus_addra/4(out29) -> bram3/1
  debus_dina/4(out29) -> bram3/2
  debus_wea/4(out29) -> bram3/3
  debus_addrb/4(out29) -> bram3/4
  debus_dinb/4(out29) -> bram3/5
  debus_web/4(out29) -> bram3/6
  debus_addra/5(out28) -> bram4/1
  debus_dina/5(out28) -> bram4/2
  debus_wea/5(out28) -> bram4/3
  debus_addrb/5(out28) -> bram4/4
  debus_dinb/5(out28) -> bram4/5
  debus_web/5(out28) -> bram4/6
  debus_addra/6(out27) -> bram5/1
  debus_dina/6(out27) -> bram5/2
  debus_wea/6(out27) -> bram5/3
  debus_addrb/6(out27) -> bram5/4
  debus_dinb/6(out27) -> bram5/5
  debus_web/6(out27) -> bram5/6
  debus_addra/7(out26) -> bram6/1
  debus_dina/7(out26) -> bram6/2
  debus_wea/7(out26) -> bram6/3
  debus_addrb/7(out26) -> bram6/4
  debus_dinb/7(out26) -> bram6/5
  debus_web/7(out26) -> bram6/6
  debus_addra/8(out25) -> bram7/1
  debus_dina/8(out25) -> bram7/2
  debus_wea/8(out25) -> bram7/3
  debus_addrb/8(out25) -> bram7/4
  debus_dinb/8(out25) -> bram7/5
  debus_web/8(out25) -> bram7/6
  debus_addra/9(out24) -> bram8/1
  debus_dina/9(out24) -> bram8/2
  debus_wea/9(out24) -> bram8/3
  debus_addrb/9(out24) -> bram8/4
  debus_dinb/9(out24) -> bram8/5
  debus_web/9(out24) -> bram8/6
  debus_addra/10(out23) -> bram9/1
  debus_dina/10(out23) -> bram9/2
  debus_wea/10(out23) -> bram9/3
  debus_addrb/10(out23) -> bram9/4
  debus_dinb/10(out23) -> bram9/5
  debus_web/10(out23) -> bram9/6
  debus_addra/11(out22) -> bram10/1
  debus_dina/11(out22) -> bram10/2
  debus_wea/11(out22) -> bram10/3
  debus_addrb/11(out22) -> bram10/4
  debus_dinb/11(out22) -> bram10/5
  debus_web/11(out22) -> bram10/6
  debus_addra/12(out21) -> bram11/1
  debus_dina/12(out21) -> bram11/2
  debus_wea/12(out21) -> bram11/3
  debus_addrb/12(out21) -> bram11/4
  debus_dinb/12(out21) -> bram11/5
  debus_web/12(out21) -> bram11/6
  debus_addra/13(out20) -> bram12/1
  debus_dina/13(out20) -> bram12/2
  debus_wea/13(out20) -> bram12/3
  debus_addrb/13(out20) -> bram12/4
  debus_dinb/13(out20) -> bram12/5
  debus_web/13(out20) -> bram12/6
  debus_addra/14(out19) -> bram13/1
  debus_dina/14(out19) -> bram13/2
  debus_wea/14(out19) -> bram13/3
  debus_addrb/14(out19) -> bram13/4
  debus_dinb/14(out19) -> bram13/5
  debus_web/14(out19) -> bram13/6
  debus_addra/15(out18) -> bram14/1
  debus_dina/15(out18) -> bram14/2
  debus_wea/15(out18) -> bram14/3
  debus_addrb/15(out18) -> bram14/4
  debus_dinb/15(out18) -> bram14/5
  debus_web/15(out18) -> bram14/6
  debus_addra/16(out17) -> bram15/1
  debus_dina/16(out17) -> bram15/2
  debus_wea/16(out17) -> bram15/3
  debus_addrb/16(out17) -> bram15/4
  debus_dinb/16(out17) -> bram15/5
  debus_web/16(out17) -> bram15/6
  debus_addra/17(out16) -> bram16/1
  debus_dina/17(out16) -> bram16/2
  debus_wea/17(out16) -> bram16/3
  debus_addrb/17(out16) -> bram16/4
  debus_dinb/17(out16) -> bram16/5
  debus_web/17(out16) -> bram16/6
  debus_addra/18(out15) -> bram17/1
  debus_dina/18(out15) -> bram17/2
  debus_wea/18(out15) -> bram17/3
  debus_addrb/18(out15) -> bram17/4
  debus_dinb/18(out15) -> bram17/5
  debus_web/18(out15) -> bram17/6
  debus_addra/19(out14) -> bram18/1
  debus_dina/19(out14) -> bram18/2
  debus_wea/19(out14) -> bram18/3
  debus_addrb/19(out14) -> bram18/4
  debus_dinb/19(out14) -> bram18/5
  debus_web/19(out14) -> bram18/6
  debus_addra/20(out13) -> bram19/1
  debus_dina/20(out13) -> bram19/2
  debus_wea/20(out13) -> bram19/3
  debus_addrb/20(out13) -> bram19/4
  debus_dinb/20(out13) -> bram19/5
  debus_web/20(out13) -> bram19/6
  debus_addra/21(out12) -> bram20/1
  debus_dina/21(out12) -> bram20/2
  debus_wea/21(out12) -> bram20/3
  debus_addrb/21(out12) -> bram20/4
  debus_dinb/21(out12) -> bram20/5
  debus_web/21(out12) -> bram20/6
  debus_addra/22(out11) -> bram21/1
  debus_dina/22(out11) -> bram21/2
  debus_wea/22(out11) -> bram21/3
  debus_addrb/22(out11) -> bram21/4
  debus_dinb/22(out11) -> bram21/5
  debus_web/22(out11) -> bram21/6
  debus_addra/23(out10) -> bram22/1
  debus_dina/23(out10) -> bram22/2
  debus_wea/23(out10) -> bram22/3
  debus_addrb/23(out10) -> bram22/4
  debus_dinb/23(out10) -> bram22/5
  debus_web/23(out10) -> bram22/6
  debus_addra/24(out9) -> bram23/1
  debus_dina/24(out9) -> bram23/2
  debus_wea/24(out9) -> bram23/3
  debus_addrb/24(out9) -> bram23/4
  debus_dinb/24(out9) -> bram23/5
  debus_web/24(out9) -> bram23/6
  debus_addra/25(out8) -> bram24/1
  debus_dina/25(out8) -> bram24/2
  debus_wea/25(out8) -> bram24/3
  debus_addrb/25(out8) -> bram24/4
  debus_dinb/25(out8) -> bram24/5
  debus_web/25(out8) -> bram24/6
  debus_addra/26(out7) -> bram25/1
  debus_dina/26(out7) -> bram25/2
  debus_wea/26(out7) -> bram25/3
  debus_addrb/26(out7) -> bram25/4
  debus_dinb/26(out7) -> bram25/5
  debus_web/26(out7) -> bram25/6
  debus_addra/27(out6) -> bram26/1
  debus_dina/27(out6) -> bram26/2
  debus_wea/27(out6) -> bram26/3
  debus_addrb/27(out6) -> bram26/4
  debus_dinb/27(out6) -> bram26/5
  debus_web/27(out6) -> bram26/6
  debus_addra/28(out5) -> bram27/1
  debus_dina/28(out5) -> bram27/2
  debus_wea/28(out5) -> bram27/3
  debus_addrb/28(out5) -> bram27/4
  debus_dinb/28(out5) -> bram27/5
  debus_web/28(out5) -> bram27/6
  debus_addra/29(out4) -> bram28/1
  debus_dina/29(out4) -> bram28/2
  debus_wea/29(out4) -> bram28/3
  debus_addrb/29(out4) -> bram28/4
  debus_dinb/29(out4) -> bram28/5
  debus_web/29(out4) -> bram28/6
  debus_addra/30(out3) -> bram29/1
  debus_dina/30(out3) -> bram29/2
  debus_wea/30(out3) -> bram29/3
  debus_addrb/30(out3) -> bram29/4
  debus_dinb/30(out3) -> bram29/5
  debus_web/30(out3) -> bram29/6
  debus_addra/31(out2) -> bram30/1
  debus_dina/31(out2) -> bram30/2
  debus_wea/31(out2) -> bram30/3
  debus_addrb/31(out2) -> bram30/4
  debus_dinb/31(out2) -> bram30/5
  debus_web/31(out2) -> bram30/6
  debus_addra/32(lsb_out1) -> bram31/1
  debus_dina/32(lsb_out1) -> bram31/2
  debus_wea/32(lsb_out1) -> bram31/3
  debus_addrb/32(lsb_out1) -> bram31/4
  debus_dinb/32(lsb_out1) -> bram31/5
  debus_web/32(lsb_out1) -> bram31/6
  bram0/1 -> A_bussify/1(in1)
  bram0/2 -> B_bussify/1(in1)
  bram1/1 -> A_bussify/2(in2)
  bram1/2 -> B_bussify/2(in2)
  bram2/1 -> A_bussify/3(in3)
  bram2/2 -> B_bussify/3(in3)
  bram3/1 -> A_bussify/4(in4)
  bram3/2 -> B_bussify/4(in4)
  bram4/1 -> A_bussify/5(in5)
  bram4/2 -> B_bussify/5(in5)
  bram5/1 -> A_bussify/6(in6)
  bram5/2 -> B_bussify/6(in6)
  bram6/1 -> A_bussify/7(in7)
  bram6/2 -> B_bussify/7(in7)
  bram7/1 -> A_bussify/8(in8)
  bram7/2 -> B_bussify/8(in8)
  bram8/1 -> A_bussify/9(in9)
  bram8/2 -> B_bussify/9(in9)
  bram9/1 -> A_bussify/10(in10)
  bram9/2 -> B_bussify/10(in10)
  bram10/1 -> A_bussify/11(in11)
  bram10/2 -> B_bussify/11(in11)
  bram11/1 -> A_bussify/12(in12)
  bram11/2 -> B_bussify/12(in12)
  bram12/1 -> A_bussify/13(in13)
  bram12/2 -> B_bussify/13(in13)
  bram13/1 -> A_bussify/14(in14)
  bram13/2 -> B_bussify/14(in14)
  bram14/1 -> A_bussify/15(in15)
  bram14/2 -> B_bussify/15(in15)
  bram15/1 -> A_bussify/16(in16)
  bram15/2 -> B_bussify/16(in16)
  bram16/1 -> A_bussify/17(in17)
  bram16/2 -> B_bussify/17(in17)
  bram17/1 -> A_bussify/18(in18)
  bram17/2 -> B_bussify/18(in18)
  bram18/1 -> A_bussify/19(in19)
  bram18/2 -> B_bussify/19(in19)
  bram19/1 -> A_bussify/20(in20)
  bram19/2 -> B_bussify/20(in20)
  bram20/1 -> A_bussify/21(in21)
  bram20/2 -> B_bussify/21(in21)
  bram21/1 -> A_bussify/22(in22)
  bram21/2 -> B_bussify/22(in22)
  bram22/1 -> A_bussify/23(in23)
  bram22/2 -> B_bussify/23(in23)
  bram23/1 -> A_bussify/24(in24)
  bram23/2 -> B_bussify/24(in24)
  bram24/1 -> A_bussify/25(in25)
  bram24/2 -> B_bussify/25(in25)
  bram25/1 -> A_bussify/26(in26)
  bram25/2 -> B_bussify/26(in26)
  bram26/1 -> A_bussify/27(in27)
  bram26/2 -> B_bussify/27(in27)
  bram27/1 -> A_bussify/28(in28)
  bram27/2 -> B_bussify/28(in28)
  bram28/1 -> A_bussify/29(in29)
  bram28/2 -> B_bussify/29(in29)
  bram29/1 -> A_bussify/30(in30)
  bram29/2 -> B_bussify/30(in30)
  bram30/1 -> A_bussify/31(in31)
  bram30/2 -> B_bussify/31(in31)
  bram31/1 -> A_bussify/32(in32)
  bram31/2 -> B_bussify/32(in32)
  A_bussify/1(bus_out) -> A/1
  B_bussify/1(bus_out) -> B/1

== system pfb_fir_generic_async_test_sim4/pfb_fir_generic/pfb_fir_taps/tap_split ==
  bus_in : Inport
  reinterpret{1..8} (8 alike) : xbsIndex_r4/Reinterpret  force_arith_type=on  arith_type=Unsigned  force_bin_pt=on  bin_pt=0  block_type=reinterpret
  slice1 : xbsIndex_r4/Slice  nbits=448  boolean_output=off  mode=Upper Bit Location + Width  bit1=-3136  base1=MSB of Input  bit0=0  base0=LSB of Input  dbl_ovrd=off  block_type=slice
  slice2 : xbsIndex_r4/Slice  nbits=448  boolean_output=off  mode=Upper Bit Location + Width  bit1=-2688  base1=MSB of Input  bit0=0  base0=LSB of Input  dbl_ovrd=off  block_type=slice
  slice3 : xbsIndex_r4/Slice  nbits=448  boolean_output=off  mode=Upper Bit Location + Width  bit1=-2240  base1=MSB of Input  bit0=0  base0=LSB of Input  dbl_ovrd=off  block_type=slice
  slice4 : xbsIndex_r4/Slice  nbits=448  boolean_output=off  mode=Upper Bit Location + Width  bit1=-1792  base1=MSB of Input  bit0=0  base0=LSB of Input  dbl_ovrd=off  block_type=slice
  slice5 : xbsIndex_r4/Slice  nbits=448  boolean_output=off  mode=Upper Bit Location + Width  bit1=-1344  base1=MSB of Input  bit0=0  base0=LSB of Input  dbl_ovrd=off  block_type=slice
  slice6 : xbsIndex_r4/Slice  nbits=448  boolean_output=off  mode=Upper Bit Location + Width  bit1=-896  base1=MSB of Input  bit0=0  base0=LSB of Input  dbl_ovrd=off  block_type=slice
  slice7 : xbsIndex_r4/Slice  nbits=448  boolean_output=off  mode=Upper Bit Location + Width  bit1=-448  base1=MSB of Input  bit0=0  base0=LSB of Input  dbl_ovrd=off  block_type=slice
  slice8 : xbsIndex_r4/Slice  nbits=448  boolean_output=off  mode=Upper Bit Location + Width  bit1=0  base1=MSB of Input  bit0=0  base0=LSB of Input  dbl_ovrd=off  block_type=slice
  msb_out8 : Outport
  out7 : Outport  Port=2
  out6 : Outport  Port=3
  out5 : Outport  Port=4
  out4 : Outport  Port=5
  out3 : Outport  Port=6
  out2 : Outport  Port=7
  lsb_out1 : Outport  Port=8
  wires:
  bus_in/1 -> slice8/1, slice7/1, slice6/1, slice5/1, slice4/1, slice3/1, slice2/1, slice1/1
  slice8/1 -> reinterpret8/1
  reinterpret8/1 -> msb_out8/1
  slice7/1 -> reinterpret7/1
  reinterpret7/1 -> out7/1
  slice6/1 -> reinterpret6/1
  reinterpret6/1 -> out6/1
  slice5/1 -> reinterpret5/1
  reinterpret5/1 -> out5/1
  slice4/1 -> reinterpret4/1
  reinterpret4/1 -> out4/1
  slice3/1 -> reinterpret3/1
  reinterpret3/1 -> out3/1
  slice2/1 -> reinterpret2/1
  reinterpret2/1 -> out2/1
  slice1/1 -> reinterpret1/1
  reinterpret1/1 -> lsb_out1/1
